simulink model "ISOP_SRCDAB"  (R2024b)
settings: Solver=VariableStepAuto  StartTime=0.0  StopTime=1  FixedStep=1e-6  RelTol=1e-3
libraries: spsSeriesRLCBranchLib x7, spsOnDelayLib x4, spsUniversalBridgeLib x4, spsCurrentMeasurementLib x2, spsLinearTransformerLib x2, spsVoltageMeasurementLib x2, spsDCVoltageSourceLib x1, sps_lib x1
settings Model: SimulationMode=accelerator  Creator=liwomin  LastModifiedBy=liwomin
settings OptimizationCC: AccelVerboseBuild=on

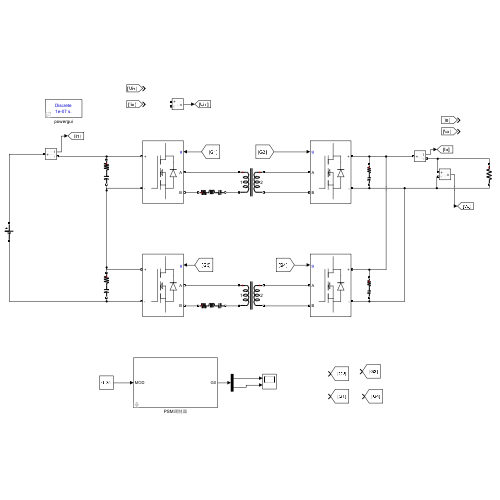
[thumbnail: Simulink's stored preview of the top-level diagram]
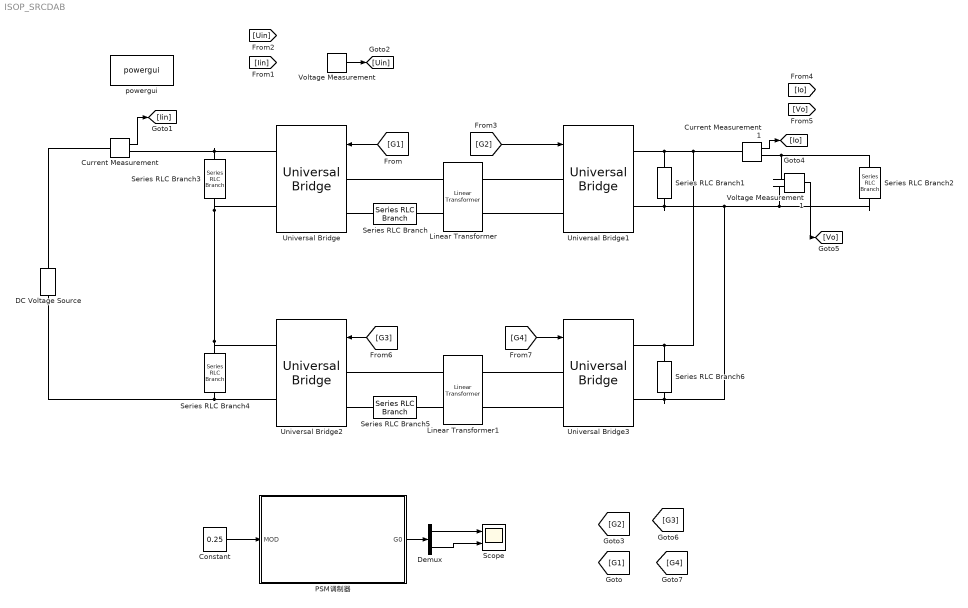
== system ISOP_SRCDAB ==
  Constant : Constant  Value=0.25
  Current Measurement : spsCurrentMeasurementLib/Current Measurement  PhasorSimulation=off  OutputType=Complex  PSBequivalent=0
  Current Measurement1 : spsCurrentMeasurementLib/Current Measurement  PhasorSimulation=off  OutputType=Complex  PSBequivalent=0
  DC Voltage Source : spsDCVoltageSourceLib/DC Voltage Source  Amplitude=400  Measurements=None
  Demux : Demux  Outputs=2
  Linear Transformer : spsLinearTransformerLib/Linear Transformer  UNITS=SI  NominalPower=[ 5000 100e3 ]  winding1=[500 0.005 0]  winding2=[100 0.005 0]  ThreeWindings=off  winding3=[3.15e+05 0.7938 0.084225]  RmLm=[1e5 3e-3]  Measurements=None  DataType=on
  Linear Transformer1 : spsLinearTransformerLib/Linear Transformer  UNITS=SI  NominalPower=[ 5000 100e3 ]  winding1=[500 0.005 0]  winding2=[100 0.005 0]  ThreeWindings=off  winding3=[3.15e+05 0.7938 0.084225]  RmLm=[1e5 3e-3]  Measurements=None  DataType=on
  PSM调制器 : Subsystem  mask{FS=100E3, DT=1E-7}
      mask DialogControl ParameterGroupVar Prompt: 参数
  Scope : Scope  NumInputPorts=2
  Series RLC Branch : spsSeriesRLCBranchLib/Series RLC Branch  LConnTagsString=__new0  RConnTagsString=__new0  BranchType=RLC  Resistance=0.005  Inductance=50e-6  SetiL0=off  InitialCurrent=0  Capacitance=100e-9  Setx0=off  InitialVoltage=0  Measurements=None
  Series RLC Branch{1,3..4,6} (4 alike) : spsSeriesRLCBranchLib/Series RLC Branch  LConnTagsString=__new0  RConnTagsString=__new0  BranchType=RC  Resistance=0.005  Inductance=1e-3  SetiL0=off  InitialCurrent=0  Capacitance=2200e-6  Setx0=off  InitialVoltage=0  Measurements=None
  Series RLC Branch2 : spsSeriesRLCBranchLib/Series RLC Branch  LConnTagsString=__new0  RConnTagsString=__new0  BranchType=R  Resistance=30  Inductance=1e-3  SetiL0=off  InitialCurrent=0  Capacitance=2200e-6  Setx0=off  InitialVoltage=0  Measurements=None
  Series RLC Branch5 : spsSeriesRLCBranchLib/Series RLC Branch  LConnTagsString=__new0  RConnTagsString=__new0  BranchType=RLC  Resistance=0.005  Inductance=50e-6  SetiL0=off  InitialCurrent=0  Capacitance=100e-9  Setx0=off  InitialVoltage=0  Measurements=None
  Universal Bridge{,1..3} (4 alike) : spsUniversalBridgeLib/Universal Bridge  Arms=2  SnubberResistance=1e5  SnubberCapacitance=inf  Device=MOSFET / Diodes  Ron=1e-3  Lon=0  ForwardVoltages="[  0  0  ]"  ForwardVoltage=0  GTOparameters=[ 10e-6 , 20e-6 ]  IGBTparameters=[ 1e-6 , 2e-6 ]  Measurements=None  Measurements_2=None  converterType=Rectifier
  Voltage Measurement : spsVoltageMeasurementLib/Voltage Measurement  PhasorSimulation=off  OutputType=Complex  PSBequivalent=0
  Voltage Measurement1 : spsVoltageMeasurementLib/Voltage Measurement  PhasorSimulation=off  OutputType=Complex  PSBequivalent=0
  powergui : sps_lib/powergui  Priority=1  SimulationMode=Discrete  SampleTime=1e-7  frequency=60  Iterations=50  frequencyindice=0  Pbase=100e6  ErrMax=1e-4  UnitsV=kV  UnitsW=MW  buscounter=0  FunctionMessages=off  echomessages=off  EnableUseOfTLC=off  CurrentSourceSwitches=off  DisableSnubberDevices=off  DisableRonSwitches=off  DisableVfSwitches=off  DisplayEquations=off  AutomaticDiscreteSolvers=off  SolverType=Tustin/Backward Euler (TBE)  Interpol=off  ExternalGateDelay=off  methode=off  Ts=100  x0status=blocks  SPID=on  SwTol=0  HookPort=off  NonlinearTolerance=1e-4  nMaxIteration=100  ContinueOnMaxIteration=off  RestoreLinks=warning  ResistiveCurrentMeasurement=off  Frange=[0:2:500]  Ylog=off  Xlog=on  ShowGrid=off  save=off  variable=ZData  structure=0  ZoomFFT=off  StartTime=0.0  cycles=1  DisplayStyle=1  fundamental=60  FreqAxis=off  MaxFrequency=1000  frequencyindicesteady=1  RmsSteady=1  display=off
  wires:
  [G1] -> Universal Bridge/1
  Current Measurement/1 -> [Iin]
  Voltage Measurement/1 -> [Uin]
  [G2] -> Universal Bridge1/1
  Current Measurement1/1 -> [Io]
  Voltage Measurement1/1 -> [Vo]
  [G3] -> Universal Bridge2/1
  [G4] -> Universal Bridge3/1
  Constant/1 -> PSM调制器/1(MOD)
  Demux/1 -> Scope/1
  PSM调制器/1(G0) -> Demux/1
  Demux/2 -> Scope/2
  connections:
  Linear Transformer/LConn2 -- Series RLC Branch/RConn1
  Universal Bridge/LConn1 -- Linear Transformer/LConn1
  Universal Bridge/LConn2 -- Series RLC Branch/LConn1
  Series RLC Branch3/RConn1 -- Series RLC Branch4/LConn1 -- Universal Bridge2/RConn1 -- Universal Bridge/RConn2
  Current Measurement/RConn1 -- Series RLC Branch3/LConn1 -- Universal Bridge/RConn1
  Current Measurement/LConn1 -- DC Voltage Source/RConn1
  Universal Bridge1/LConn1 -- Linear Transformer/RConn1
  Universal Bridge1/LConn2 -- Linear Transformer/RConn2
  Current Measurement1/RConn1 -- Voltage Measurement1/LConn1 -- Series RLC Branch2/LConn1
  Series RLC Branch2/RConn1 -- Voltage Measurement1/LConn2 -- Series RLC Branch6/RConn1 -- Universal Bridge3/RConn2 -- Series RLC Branch1/RConn1 -- Universal Bridge1/RConn2
  Universal Bridge1/RConn1 -- Series RLC Branch1/LConn1 -- Series RLC Branch6/LConn1 -- Universal Bridge3/RConn1 -- Current Measurement1/LConn1
  Universal Bridge2/RConn2 -- DC Voltage Source/LConn1 -- Series RLC Branch4/RConn1
  Linear Transformer1/LConn1 -- Universal Bridge2/LConn1
  Series RLC Branch5/RConn1 -- Linear Transformer1/LConn2
  Series RLC Branch5/LConn1 -- Universal Bridge2/LConn2
  Universal Bridge3/LConn1 -- Linear Transformer1/RConn1
  Universal Bridge3/LConn2 -- Linear Transformer1/RConn2

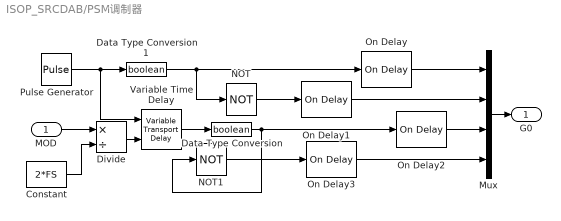
== system ISOP_SRCDAB/PSM调制器 ==
  MOD : Inport
  Constant : Constant  Value=2*FS  VectorParams1D=off
  Data Type Conversion : DataTypeConversion  OutDataTypeStr=boolean  SaturateOnIntegerOverflow=off  RndMeth=Floor
  Data Type Conversion1 : DataTypeConversion  OutDataTypeStr=boolean  SaturateOnIntegerOverflow=off  RndMeth=Floor
  Divide : Product  Inputs=*/
  Mux : Mux
  NOT : Logic  Operator=NOT  IconShape=distinctive  AllPortsSameDT=off  OutDataTypeStr=boolean
  NOT1 : Logic  Operator=NOT  IconShape=distinctive  AllPortsSameDT=off  OutDataTypeStr=boolean
  On Delay{,1..3} (4 alike) : spsOnDelayLib/On Delay  DelayType=On delay  delay=DT  ic=0  Ts=0
  Pulse Generator : DiscretePulseGenerator  PulseType=Time based  Period=1/FS  PulseWidth=50
  Variable Time Delay : VariableTransportDelay  MaximumDelay=10
  G0 : Outport
  wires:
  Data Type Conversion1/1 -> On Delay/1, NOT/1
  Pulse Generator/1 -> Data Type Conversion1/1, Variable Time Delay/1
  Constant/1 -> Divide/2
  MOD/1 -> Divide/1
  Divide/1 -> Variable Time Delay/2
  NOT1/1 -> On Delay3/1
  Data Type Conversion/1 -> On Delay2/1, NOT1/1
  Variable Time Delay/1 -> Data Type Conversion/1
  Mux/1 -> G0/1
  NOT/1 -> On Delay1/1
  On Delay/1 -> Mux/1
  On Delay1/1 -> Mux/2
  On Delay2/1 -> Mux/3
  On Delay3/1 -> Mux/4
